simulink model "testBlockDiff"  (R2023b)
settings: Solver=VariableStepAuto  StartTime=0.0  StopTime=10.0  RelTol=1e-3
libraries: visionhdlconversions x1, matrix_library x1
settings Model: Creator=neham  LastModifiedBy=neham

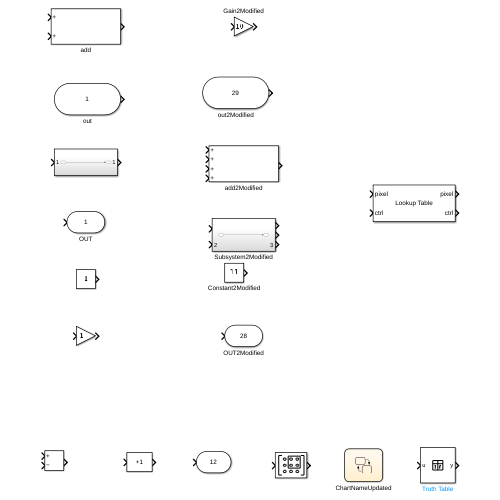
[thumbnail: Simulink's stored preview of the top-level diagram]
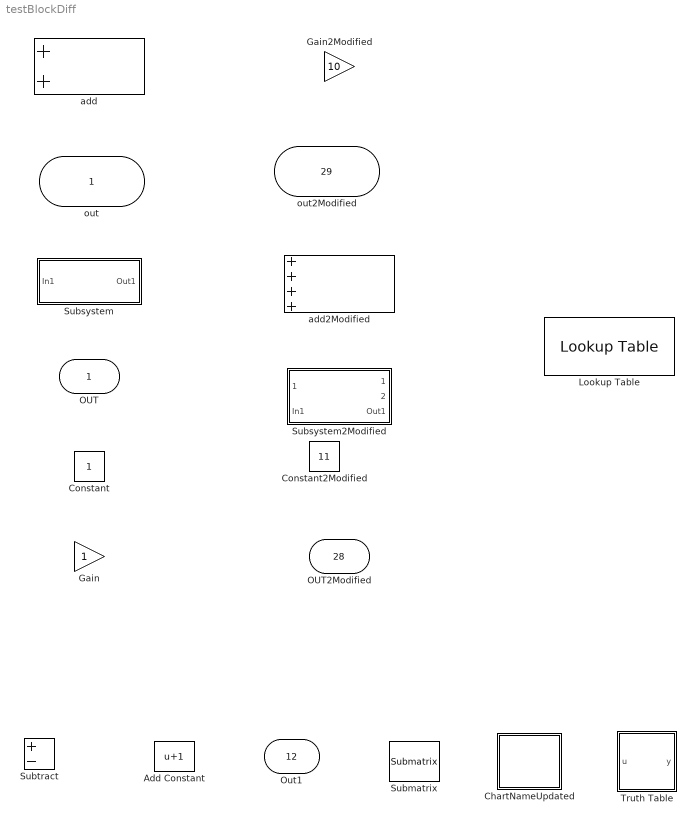
== system testBlockDiff ==
  out : Inport
  out2Modified : Inport  Port=29
  Add Constant : Bias  Bias=1  SaturateOnIntegerOverflow=off
  ChartNameUpdated : Stateflow chart  TreatAsAtomicUnit=on
  Constant : Constant
  Constant2Modified : Constant  Value=11
  Gain : Gain
  Gain2Modified : Gain  Gain=10
  Lookup Table : visionhdlconversions/Lookup Table  Table=uint8( 0:1:255 )  SimulateUsing=Code generation
  Submatrix : matrix_library/Submatrix  RowSpan=Range of rows  RowStartMode=First  RowStartIndex=1  RowEndMode=Last  RowEndIndex=1  ColSpan=Range of columns  ColStartMode=First  ColStartIndex=1  ColEndMode=Last  ColEndIndex=1
  Subsystem : Subsystem
  Subsystem2Modified : Subsystem
  Subtract : Sum  Inputs=+-
  Truth Table : Truth Table  TreatAsAtomicUnit=on
  add : Sum
  add2Modified : Sum  Inputs=++++
  OUT : Outport
  Out1 : Outport  Port=12  VectorParamsAs1DForOutWhenUnconnected=off
  OUT2Modified : Outport  Port=28

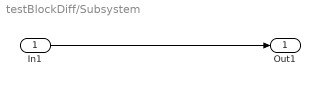
== system testBlockDiff/Subsystem ==
  In1 : Inport
  Out1 : Outport
  wires:
  In1/1 -> Out1/1

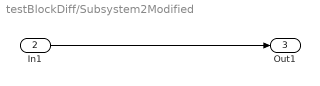
== system testBlockDiff/Subsystem2Modified ==
  In1 : Inport  Port=2
  Out1 : Outport  Port=3
  wires:
  In1/1 -> Out1/1

== stateflow chart testBlockDiff/ChartNameUpdated ==

== matlab function testBlockDiff/Truth Table ==
  data: u input; y output
function y = fcn(u)

aVarTruthTableCondition_1 = false;
aVarTruthTableCondition_2 = false;


% Example condition 1

aVarTruthTableCondition_1 = logical(u >= 0);

% Example condition 2

aVarTruthTableCondition_2 = logical(u ^ 2 <= 1);

if (aVarTruthTableCondition_1 && aVarTruthTableCondition_2)
    aFcnTruthTableAction_1();
elseif (~aVarTruthTableCondition_1 && ~aVarTruthTableCondition_2)
    aFcnTruthTableAction_1();
else % Default
    aFcnTruthTableAction_2();
end

function aFcnTruthTableAction_1()

% Example action 1 called from D1 & D2 column in condition table

y = u;

function aFcnTruthTableAction_2()

% Example action 2 called from D3 column in condition table

y = 1 / u;
